simulink subsystem "Steer_Module_Offset_Adjustments_sub"  (R2023b)
settings: Solver=VariableStepAuto  StartTime=0.0  StopTime=10.0  RelTol=1e-3
libraries: Controls_Components_lib x4
settings Model: Creator=ander  LastModifiedBy=ander

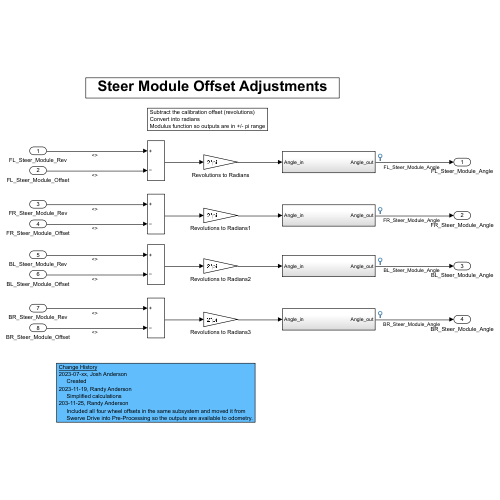
[thumbnail: Simulink's stored preview of the top-level diagram]
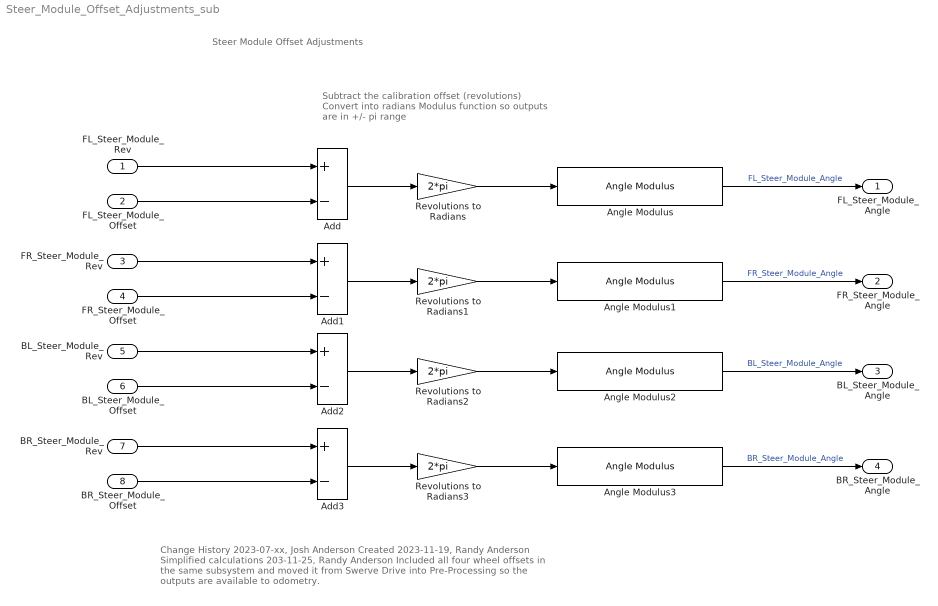
== system Steer_Module_Offset_Adjustments_sub ==
  note: Change History
      | 2023-07-xx, Josh Anderson
      | Created
      | 2023-11-19, Randy Anderson
      | Simplified calculations
      | 203-11-25, Randy Anderson
      | Included all four wheel offsets in the same subsystem and moved it from
      | Swerve Drive into Pre-Processing so the outputs are available to odometry.
  note: Subtract the calibration offset (revolutions)
      | Convert into radians
      | Modulus function so outputs are in +/- pi range
  note: Steer Module Offset Adjustments
  FL_Steer_Module_Rev : Inport  OutDataTypeStr=double  Unit=rev
  FL_Steer_Module_Offset : Inport  Port=2  OutDataTypeStr=double  Unit=rev
  FR_Steer_Module_Rev : Inport  Port=3  OutDataTypeStr=double  Unit=rev
  FR_Steer_Module_Offset : Inport  Port=4  OutDataTypeStr=double  Unit=rev
  BL_Steer_Module_Rev : Inport  Port=5  OutDataTypeStr=double  Unit=rev
  BL_Steer_Module_Offset : Inport  Port=6  OutDataTypeStr=double  Unit=rev
  BR_Steer_Module_Rev : Inport  Port=7  OutDataTypeStr=double  Unit=rev
  BR_Steer_Module_Offset : Inport  Port=8  OutDataTypeStr=double  Unit=rev
  Add{,1..3} (4 alike) : Sum  Inputs=+-
  Angle Modulus{,1..3} (4 alike) : Controls_Components_lib/Angle Modulus  SystemSampleTime=-1  VariantActivationTime=update diagram  AllowFlexibleInterface=on  Latency=0  AutoFrameSizeCalculation=off
  Revolutions to Radians{,1..3} (4 alike) : Gain  Gain=2*pi
  FL_Steer_Module_Angle : Outport  OutDataTypeStr=double  Unit=rad
  FR_Steer_Module_Angle : Outport  Port=2  OutDataTypeStr=double  Unit=rad
  BL_Steer_Module_Angle : Outport  Port=3  OutDataTypeStr=double  Unit=rad
  BR_Steer_Module_Angle : Outport  Port=4  OutDataTypeStr=double  Unit=rad
  wires:
  Add/1 -> Revolutions to Radians/1
  FL_Steer_Module_Offset/1 -> Add/2
  FL_Steer_Module_Rev/1 -> Add/1
  Revolutions to Radians/1 -> Angle Modulus/1
  FR_Steer_Module_Rev/1 -> Add1/1
  FR_Steer_Module_Offset/1 -> Add1/2
  Revolutions to Radians1/1 -> Angle Modulus1/1
  Add1/1 -> Revolutions to Radians1/1
  BL_Steer_Module_Offset/1 -> Add2/2
  BL_Steer_Module_Rev/1 -> Add2/1
  Add2/1 -> Revolutions to Radians2/1
  Revolutions to Radians2/1 -> Angle Modulus2/1
  BR_Steer_Module_Offset/1 -> Add3/2
  BR_Steer_Module_Rev/1 -> Add3/1
  Add3/1 -> Revolutions to Radians3/1
  Revolutions to Radians3/1 -> Angle Modulus3/1
  Angle Modulus/1 -> FL_Steer_Module_Angle/1  "FL_Steer_Module_Angle"
  Angle Modulus1/1 -> FR_Steer_Module_Angle/1  "FR_Steer_Module_Angle"
  Angle Modulus2/1 -> BL_Steer_Module_Angle/1  "BL_Steer_Module_Angle"
  Angle Modulus3/1 -> BR_Steer_Module_Angle/1  "BR_Steer_Module_Angle"
